simulink model "Diesel_Genset_Test_System"  (Simulink 8.1)
settings: Solver=ode3  SolverMode=SingleTasking  StartTime=0.0  StopTime=150  FixedStep=Ts  RelTol=1e-3
PostLoadFcn:
  | Ts=50e-6;SIM_HIL=0;
InitFcn:
  | Ts=50e-6;SIM_HIL=0;
undefined symbols (not defined in the file): Gen_900kW_external_control, HIL_GenSet, Left, type, V
libraries: powerlib x31, powerlib_extras x24, simulink x10, dspsigops x6, breakers_1ph_3ph x6, rtio_generic_modbus x6, cables_lib x5, rtlab x2, ssn_lib x2, artemis x1, Diesel_Genset_lib x1
(part 2 of 3)

== system Diesel_Genset_Test_System/SM_Master/MODBUS8 ==
  note: S commands:
      | S: 0 , for logic operated relays
      | S: 1 ,  for remotely close the breaker unit
      | S: 2 , for remotely open the breaker unit
  Op_Mode : Inport
  Bus Creator : BusCreator  Inputs=2
  Data Type Conversion1 : DataTypeConversion
  Delay1 : dspsigops/Delay  dly_unit=Samples  delay=lower((3/60)/Ts)  ic_detail=off  dif_ic_for_ch=off  dif_ic_for_dly=off  ic=1  reset_popup=None
  Ground : powerlib/Elements/Ground  LConnTagsString=a
  Index Vector : MultiPortSwitch  DataPortOrder=Zero-based contiguous  DataPortIndices={2,1,0}  zeroidx=on
  SEL_787_Relay : Subsystem
  Three-Phase Parallel RLC Branch : powerlib/Elements/Three-Phase Parallel RLC Branch  LConnTagsString=A|B|C  RConnTagsString=A|B|C  BranchType=R  Resistance=10e6  Inductance=1e-3  Capacitance=1e-6  Measurements=None
  Three-Phase V-I Measurement : powerlib/Measurements/Three-Phase V-I Measurement  VoltageMeasurement=phase-to-ground  SetLabelV=off  LabelV=Vabc  Vpu=off  VpuLL=off  CurrentMeasurement=yes  SetLabelI=off  LabelI=Iabc  Ipu=off  Pbase=100e6  Vbase=500e3  OutputType=Complex  PhasorSimulation=off  PSBequivalent=0
  Three-Phase Breaker : powerlib/Elements/Three-Phase Breaker  InitialState=open  SwitchA=on  SwitchB=on  SwitchC=on  SwitchTimes="[1/60  5/60]"  External=on  BreakerResistance=1e-3  SnubberResistance=0  SnubberCapacitance=0  Measurements=None
  close : Constant
  open : Constant  Value=0
  A : PMIOPort  Tag=PMCPort  Port=1  Side=Left
  B : PMIOPort  Tag=PMCPort  Port=2  Side=Left
  C : PMIOPort  Tag=PMCPort  Port=3  Side=Left
  a : PMIOPort  Tag=PMCPort  Port=4  Side=Right
  b : PMIOPort  Tag=PMCPort  Port=5  Side=Right
  c : PMIOPort  Tag=PMCPort  Port=6  Side=Right
  m : Outport
  wires:
  [m] -> Bus Creator/2  "sel_787"
  SEL_787_Relay/3(m) -> [m]
  Bus Creator/1 -> m/1  "m"
  [Status] -> Bus Creator/1  "Grid_Status"
  Delay1/1 -> [Status], Three-Phase Breaker/1
  Three-Phase V-I Measurement/1 -> [Vabc]
  Three-Phase V-I Measurement/2 -> [Iabc]
  open/1 -> Index Vector/4
  close/1 -> Index Vector/3
  Index Vector/1 -> Data Type Conversion1/1
  Data Type Conversion1/1 -> Delay1/1
  [Iabc] -> SEL_787_Relay/1(Iabc_w1)  "Iabc"
  [Vabc] -> SEL_787_Relay/2(Vabc)  "Vabc"
  SEL_787_Relay/2(Logic_trip) -> Index Vector/2
  Op_Mode/1 -> Index Vector/1
  connections:
  Three-Phase V-I Measurement/RConn1 -- Three-Phase Parallel RLC Branch/RConn1 -- Three-Phase Breaker/LConn1
  Three-Phase V-I Measurement/RConn2 -- Three-Phase Parallel RLC Branch/RConn2 -- Three-Phase Breaker/LConn2
  Three-Phase V-I Measurement/RConn3 -- Three-Phase Parallel RLC Branch/RConn3 -- Three-Phase Breaker/LConn3
  Three-Phase Breaker/RConn2 -- b/RConn1
  Three-Phase Breaker/RConn3 -- c/RConn1
  Three-Phase V-I Measurement/LConn1 -- A/RConn1
  a/RConn1 -- Three-Phase Breaker/RConn1
  C/RConn1 -- Three-Phase V-I Measurement/LConn3
  B/RConn1 -- Three-Phase V-I Measurement/LConn2
  Ground/LConn1 -- Three-Phase Parallel RLC Branch/LConn2 -- Three-Phase Parallel RLC Branch/LConn3 -- Three-Phase Parallel RLC Branch/LConn1

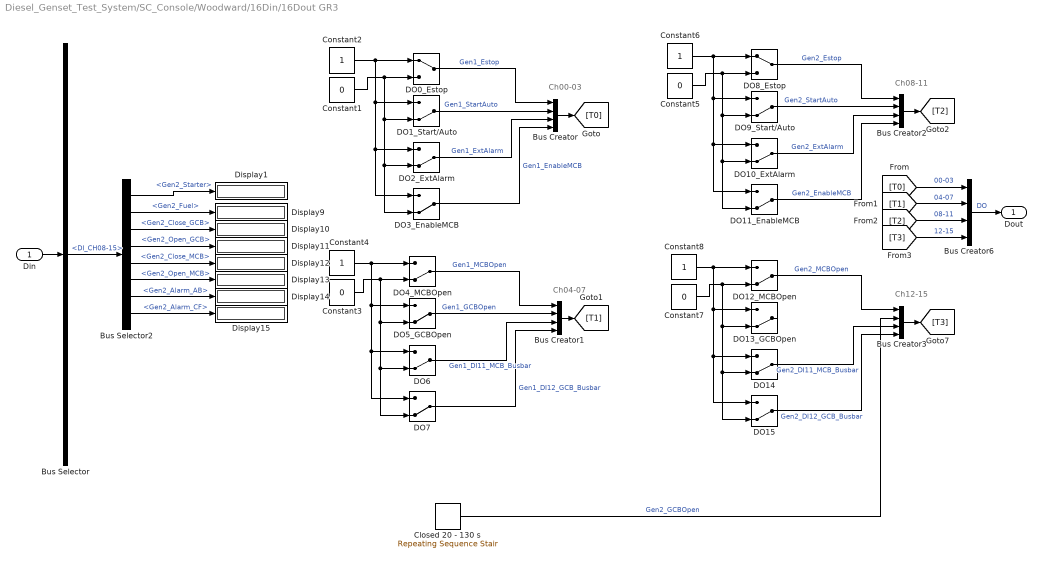
== system Diesel_Genset_Test_System/SC_Console/Woodward/16Din/16Dout GR3 ==
  note: Ch00-03
  note: Ch04-07
  note: Ch08-11
  note: Ch12-15
  Din : Inport
  Bus Creator{,1..3,6} (5 alike) : BusCreator
  Bus Selector : BusSelector  OutputSignals=DIN.DI_CH08-15
  Bus Selector2 : BusSelector  OutputSignals=Gen2_Starter,Gen2_Fuel,Gen2_Close_GCB,Gen2_Open_GCB,Gen2_Close_MCB,Gen2_Open_MCB,Gen2_Alarm_AB,Gen2_Alarm_CF
  Closed 20 - 130 s : simulink/Sources/Repeating Sequence Stair  OutValues=[1 1 1 1 0 0 0 0 0 0 0 0 0 0 0 0 0 0 0 0 0 0 0 0 0 0 1 1 1 1 1 ]  tsamp=[5 Ts]  OutMin=[]  OutMax=[]  OutDataTypeStr=double  OutputDataTypeScalingMode=double  OutDataType=fixdt(0,8)  ConRadixGroup=Best Precision: Vector-wise  OutScaling=2^-12
  Constant{1,3,5,7} (4 alike) : Constant  Value=0
  Constant{2,4,6,8} (4 alike) : Constant
  DO0_Estop : ManualSwitch
  DO10_ExtAlarm : ManualSwitch  CurrentSetting=0
  DO11_EnableMCB : ManualSwitch  CurrentSetting=0
  DO12_MCBOpen : ManualSwitch  CurrentSetting=0
  DO13_GCBOpen : ManualSwitch  CurrentSetting=0
  DO{6..7,14..15} (4 alike) : ManualSwitch  CurrentSetting=0
  DO1_Start/Auto : ManualSwitch  CurrentSetting=0
  DO2_ExtAlarm : ManualSwitch  CurrentSetting=0
  DO3_EnableMCB : ManualSwitch  CurrentSetting=0
  DO4_MCBOpen : ManualSwitch  CurrentSetting=0
  DO5_GCBOpen : ManualSwitch  CurrentSetting=0
  DO8_Estop : ManualSwitch
  DO9_Start/Auto : ManualSwitch  CurrentSetting=0
  Display{1,9..15} (8 alike) : Display
  Dout : Outport
  wires:
  Bus Creator6/1 -> Dout/1  "DO"
  Constant2/1 -> DO0_Estop/1, DO1_Start/Auto/1, DO3_EnableMCB/1, DO2_ExtAlarm/1
  Constant1/1 -> DO0_Estop/2, DO1_Start/Auto/2, DO3_EnableMCB/2, DO2_ExtAlarm/2
  DO0_Estop/1 -> Bus Creator/1  "Gen1_Estop"
  DO1_Start/Auto/1 -> Bus Creator/2  "Gen1_StartAuto"
  DO2_ExtAlarm/1 -> Bus Creator/3  "Gen1_ExtAlarm"
  DO3_EnableMCB/1 -> Bus Creator/4  "Gen1_EnableMCB"
  Constant4/1 -> DO6/1, DO7/1, DO5_GCBOpen/1, DO4_MCBOpen/1
  Constant3/1 -> DO6/2, DO7/2, DO5_GCBOpen/2, DO4_MCBOpen/2
  DO4_MCBOpen/1 -> Bus Creator1/1  "Gen1_MCBOpen"
  DO6/1 -> Bus Creator1/3  "Gen1_DI11_MCB_Busbar"
  DO7/1 -> Bus Creator1/4  "Gen1_DI12_GCB_Busbar"
  Constant6/1 -> DO8_Estop/1, DO9_Start/Auto/1, DO11_EnableMCB/1, DO10_ExtAlarm/1
  Constant5/1 -> DO8_Estop/2, DO9_Start/Auto/2, DO11_EnableMCB/2, DO10_ExtAlarm/2
  DO8_Estop/1 -> Bus Creator2/1  "Gen2_Estop"
  DO9_Start/Auto/1 -> Bus Creator2/2  "Gen2_StartAuto"
  DO10_ExtAlarm/1 -> Bus Creator2/3  "Gen2_ExtAlarm"
  DO11_EnableMCB/1 -> Bus Creator2/4  "Gen2_EnableMCB"
  Constant8/1 -> DO14/1, DO15/1, DO13_GCBOpen/1, DO12_MCBOpen/1
  Constant7/1 -> DO14/2, DO15/2, DO13_GCBOpen/2, DO12_MCBOpen/2
  DO12_MCBOpen/1 -> Bus Creator3/1  "Gen2_MCBOpen"
  DO14/1 -> Bus Creator3/3  "Gen2_DI11_MCB_Busbar"
  DO15/1 -> Bus Creator3/4  "Gen2_DI12_GCB_Busbar"
  Bus Creator/1 -> [T0]
  Bus Creator1/1 -> [T1]
  Bus Creator3/1 -> [T3]
  Bus Creator2/1 -> [T2]
  [T0] -> Bus Creator6/1  "00-03"
  [T1] -> Bus Creator6/2  "04-07"
  [T2] -> Bus Creator6/3  "08-11"
  [T3] -> Bus Creator6/4  "12-15"
  Din/1 -> Bus Selector/1
  Bus Selector/1 -> Bus Selector2/1  "<DI_CH08-15>"
  Bus Selector2/1 -> Display1/1  "<Gen2_Starter>"
  Bus Selector2/2 -> Display9/1  "<Gen2_Fuel>"
  Bus Selector2/3 -> Display10/1  "<Gen2_Close_GCB>"
  Bus Selector2/4 -> Display11/1  "<Gen2_Open_GCB>"
  Bus Selector2/5 -> Display12/1  "<Gen2_Close_MCB>"
  Bus Selector2/6 -> Display13/1  "<Gen2_Open_MCB>"
  Bus Selector2/7 -> Display14/1  "<Gen2_Alarm_AB>"
  Bus Selector2/8 -> Display15/1  "<Gen2_Alarm_CF>"
  DO5_GCBOpen/1 -> Bus Creator1/2  "Gen1_GCBOpen"
  Closed 20 - 130 s/1 -> Bus Creator3/2  "Gen2_GCBOpen"

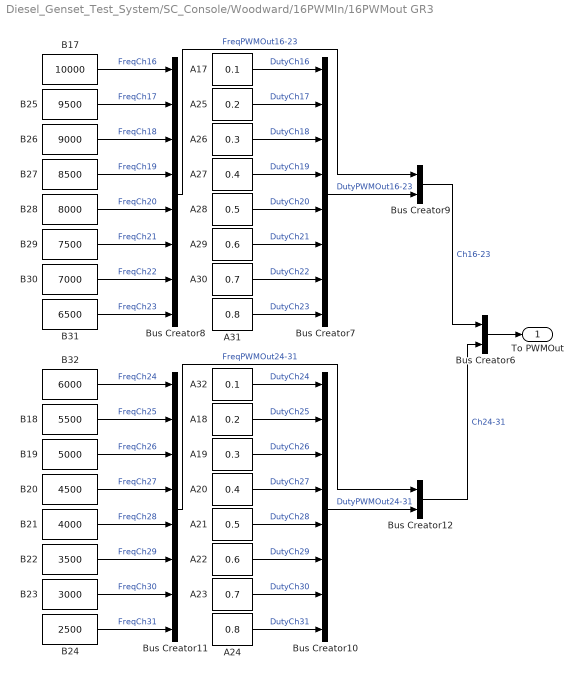
== system Diesel_Genset_Test_System/SC_Console/Woodward/16PWMIn/16PWMout GR3 ==
  A17 : Constant  Value=0.1
  A18 : Constant  Value=0.2
  A19 : Constant  Value=0.3
  A20 : Constant  Value=0.4
  A21 : Constant  Value=0.5
  A22 : Constant  Value=0.6
  A23 : Constant  Value=0.7
  A24 : Constant  Value=0.8
  A25 : Constant  Value=0.2
  A26 : Constant  Value=0.3
  A27 : Constant  Value=0.4
  A28 : Constant  Value=0.5
  A29 : Constant  Value=0.6
  A30 : Constant  Value=0.7
  A31 : Constant  Value=0.8
  A32 : Constant  Value=0.1
  B17 : Constant  Value=10000
  B18 : Constant  Value=5500
  B19 : Constant  Value=5000
  B20 : Constant  Value=4500
  B21 : Constant  Value=4000
  B22 : Constant  Value=3500
  B23 : Constant  Value=3000
  B24 : Constant  Value=2500
  B25 : Constant  Value=9500
  B26 : Constant  Value=9000
  B27 : Constant  Value=8500
  B28 : Constant  Value=8000
  B29 : Constant  Value=7500
  B30 : Constant  Value=7000
  B31 : Constant  Value=6500
  B32 : Constant  Value=6000
  Bus Creator{7..8,10..11} (4 alike) : BusCreator  Inputs=8
  Bus Creator12 : BusCreator  Inputs=2
  Bus Creator6 : BusCreator  Inputs=2
  Bus Creator9 : BusCreator  Inputs=2
  To PWMOut : Outport
  wires:
  Bus Creator6/1 -> To PWMOut/1
  A17/1 -> Bus Creator7/1  "DutyCh16"
  A25/1 -> Bus Creator7/2  "DutyCh17"
  A26/1 -> Bus Creator7/3  "DutyCh18"
  A27/1 -> Bus Creator7/4  "DutyCh19"
  A28/1 -> Bus Creator7/5  "DutyCh20"
  A29/1 -> Bus Creator7/6  "DutyCh21"
  A30/1 -> Bus Creator7/7  "DutyCh22"
  A31/1 -> Bus Creator7/8  "DutyCh23"
  B17/1 -> Bus Creator8/1  "FreqCh16"
  B25/1 -> Bus Creator8/2  "FreqCh17"
  B26/1 -> Bus Creator8/3  "FreqCh18"
  B27/1 -> Bus Creator8/4  "FreqCh19"
  B28/1 -> Bus Creator8/5  "FreqCh20"
  B29/1 -> Bus Creator8/6  "FreqCh21"
  B30/1 -> Bus Creator8/7  "FreqCh22"
  B31/1 -> Bus Creator8/8  "FreqCh23"
  Bus Creator7/1 -> Bus Creator9/2  "DutyPWMOut16-23"
  Bus Creator8/1 -> Bus Creator9/1  "FreqPWMOut16-23"
  A32/1 -> Bus Creator10/1  "DutyCh24"
  A18/1 -> Bus Creator10/2  "DutyCh25"
  A19/1 -> Bus Creator10/3  "DutyCh26"
  A20/1 -> Bus Creator10/4  "DutyCh27"
  A21/1 -> Bus Creator10/5  "DutyCh28"
  A22/1 -> Bus Creator10/6  "DutyCh29"
  A23/1 -> Bus Creator10/7  "DutyCh30"
  A24/1 -> Bus Creator10/8  "DutyCh31"
  B32/1 -> Bus Creator11/1  "FreqCh24"
  B18/1 -> Bus Creator11/2  "FreqCh25"
  B19/1 -> Bus Creator11/3  "FreqCh26"
  B20/1 -> Bus Creator11/4  "FreqCh27"
  B21/1 -> Bus Creator11/5  "FreqCh28"
  B22/1 -> Bus Creator11/6  "FreqCh29"
  B23/1 -> Bus Creator11/7  "FreqCh30"
  B24/1 -> Bus Creator11/8  "FreqCh31"
  Bus Creator10/1 -> Bus Creator12/2  "DutyPWMOut24-31"
  Bus Creator11/1 -> Bus Creator12/1  "FreqPWMOut24-31"
  Bus Creator12/1 -> Bus Creator6/2  "Ch24-31"
  Bus Creator9/1 -> Bus Creator6/1  "Ch16-23"

== system Diesel_Genset_Test_System/SC_Console/Woodward/16TSDIn/16 TSDOut GR3 ==
  Bus Creator1 : BusCreator  Inputs=3
  Din/Dout ch16-23 : Subsystem
  Din/Dout ch24-31 : Subsystem
  Dout state ctrl : Subsystem
  TSDout : Outport
  wires:
  Din/Dout ch24-31/1(Out1) -> Bus Creator1/2  "times CH24-31"
  Din/Dout ch16-23/1(Out1) -> Bus Creator1/1  "times CH16-23"
  Dout state ctrl/1(Event State OUT) -> Bus Creator1/3  "states"
  Bus Creator1/1 -> TSDout/1

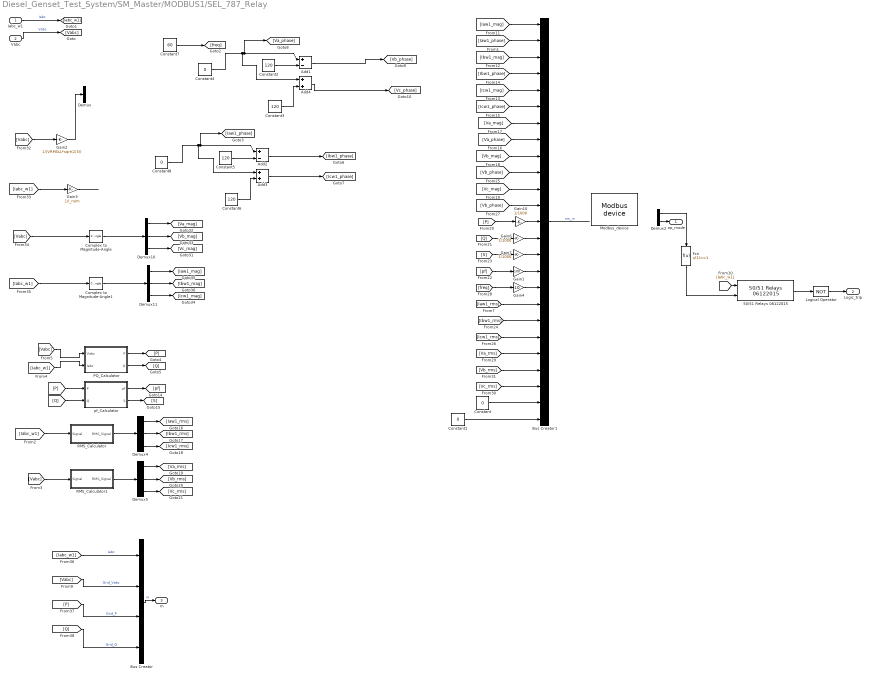
== system Diesel_Genset_Test_System/SM_Master/MODBUS1/SEL_787_Relay ==
  Iabc_w1 : Inport
  Vabc : Inport  Port=2
  50/51 Relays 06122015 : breakers_1ph_3ph/50//51 Relays 06122015  TOC=TOC  IOC=IOC  Ts=Ts
  Add1 : Sum  Inputs=+-
  Add2 : Sum  Inputs=+-
  Add3 : Sum
  Add4 : Sum
  Bus Creator : BusCreator
  Bus Creator1 : BusCreator  Inputs=25
  Complex to Magnitude-Angle : ComplexToMagnitudeAngle  Output=Magnitude
  Complex to Magnitude-Angle1 : ComplexToMagnitudeAngle  Output=Magnitude
  Constant{,1,4,8} (4 alike) : Constant  Value=0
  Constant{2..3,5..6} (4 alike) : Constant  Value=120
  Constant7 : Constant  Value=60
  Demux{,4..5,10..11} (5 alike) : Demux  Outputs=3
  Demux2 : Demux  Outputs=2
  Fcn : Fcn  Expr=u(1)==1
  Gain1 : Gain  Gain=100
  Gain10 : Gain  Gain=1/1000
  Gain2 : Gain  Gain=1/(VRMSLL*sqrt(2/3))
  Gain3 : Gain  Gain=1/I_nom
  Gain4 : Gain  Gain=10
  Gain6 : Gain  Gain=1/1000
  Gain7 : Gain  Gain=1/1000
  Logical Operator : Logic  Operator=NOT  AllPortsSameDT=off  OutDataTypeStr=boolean
  Modbus_device : rtio_generic_modbus/Modbus device  conf_name=none  conf_name_mask=relay_slave_cfg1.xls  sample_time=Ts
  PQ_Calculator : Subsystem
  RMS_Calculator : Subsystem
  RMS_Calculator1 : Subsystem
  pf_Calculator : Subsystem
  op_mode : Outport
  Logic_trip : Outport  Port=2
  m : Outport  Port=3
  wires:
  Gain4/1 -> Bus Creator1/17
  Gain1/1 -> Bus Creator1/16
  [pf] -> Gain1/1
  [freq] -> Gain4/1
  Constant4/1 -> Add4/1, [Va_phase], Add1/1
  Add4/1 -> [Vc_phase]
  Add1/1 -> [Vb_phase]
  Constant3/1 -> Add4/2
  Constant2/1 -> Add1/2
  Constant8/1 -> Add3/1, [Iaw1_phase], Add2/1
  Add3/1 -> [Icw1_phase]
  Add2/1 -> [Ibw1_phase]
  Constant6/1 -> Add3/2
  Constant5/1 -> Add2/2
  Constant7/1 -> [freq]
  pf_Calculator/2(S) -> [S]
  Bus Creator1/1 -> ?  "sm_in"
  ? -> Demux2/1
  [Q] -> Bus Creator/4  "Grid_Q"
  [P] -> Bus Creator/3  "Grid_P"
  [Vabc] -> Bus Creator/2  "Grid_Vabc"
  [Iabc_w1] -> Bus Creator/1  "Iabc"
  Bus Creator/1 -> m/1  "m"
  Iabc_w1/1 -> [Iabc_w1]  "Iabc"
  Vabc/1 -> [Vabc]  "Vabc"
  [Vabc] -> PQ_Calculator/1(Vabc)
  [Iabc_w1] -> PQ_Calculator/2(Iabc)
  [Iaw1_mag] -> Bus Creator1/1
  [P] -> Gain10/1
  [Q] -> Gain6/1
  [S] -> Gain7/1
  pf_Calculator/1(pf) -> [pf]
  [P] -> pf_Calculator/1(P)
  [Q] -> pf_Calculator/2(Q)
  PQ_Calculator/1(P) -> [P]
  PQ_Calculator/2(Q) -> [Q]
  [Iabc_w1] -> RMS_Calculator/1(Signal)
  [Vabc] -> RMS_Calculator1/1(Signal)
  RMS_Calculator/1(RMS_Signal) -> Demux4/1
  RMS_Calculator1/1(RMS_Signal) -> Demux5/1
  Demux4/3 -> [Icw1_rms]
  Demux4/2 -> [Ibw1_rms]
  Demux4/1 -> [Iaw1_rms]
  Demux5/1 -> [Va_rms]
  Demux5/2 -> [Vb_rms]
  Demux5/3 -> [Vc_rms]
  Demux2/1 -> Fcn/1
  Fcn/1 -> 50/51 Relays 06122015/2
  [Iabc_w1] -> 50/51 Relays 06122015/1
  50/51 Relays 06122015/1 -> Logical Operator/1
  [Ibw1_mag] -> Bus Creator1/3
  [Icw1_mag] -> Bus Creator1/5
  [Va_mag] -> Bus Creator1/7
  [Vb_mag] -> Bus Creator1/9
  [Vc_mag] -> Bus Creator1/11
  Gain10/1 -> Bus Creator1/13
  Gain6/1 -> Bus Creator1/14
  Gain7/1 -> Bus Creator1/15
  [Iaw1_rms] -> Bus Creator1/18
  [Icw1_rms] -> Bus Creator1/20
  [Ibw1_rms] -> Bus Creator1/19
  [Va_rms] -> Bus Creator1/21
  [Vb_rms] -> Bus Creator1/22
  [Vc_rms] -> Bus Creator1/23
  Logical Operator/1 -> Logic_trip/1
  Demux2/2 -> op_mode/1
  [Iaw1_phase] -> Bus Creator1/2
  [Ibw1_phase] -> Bus Creator1/4
  [Icw1_phase] -> Bus Creator1/6
  [Va_phase] -> Bus Creator1/8
  [Vb_phase] -> Bus Creator1/10
  [Vb_phase] -> Bus Creator1/12
  Constant/1 -> Bus Creator1/24
  Constant1/1 -> Bus Creator1/25
  [Vabc] -> Gain2/1
  Gain2/1 -> Demux/1
  [Iabc_w1] -> Gain3/1
  Gain3/1 -> ?
  Demux10/1 -> [Va_mag]
  Demux10/2 -> [Vb_mag]
  Demux10/3 -> [Vc_mag]
  Complex to Magnitude-Angle/1 -> Demux10/1
  [Vabc] -> Complex to Magnitude-Angle/1
  Complex to Magnitude-Angle1/1 -> Demux11/1
  [Iabc_w1] -> Complex to Magnitude-Angle1/1
  Demux11/1 -> [Iaw1_mag]
  Demux11/2 -> [Ibw1_mag]
  Demux11/3 -> [Icw1_mag]

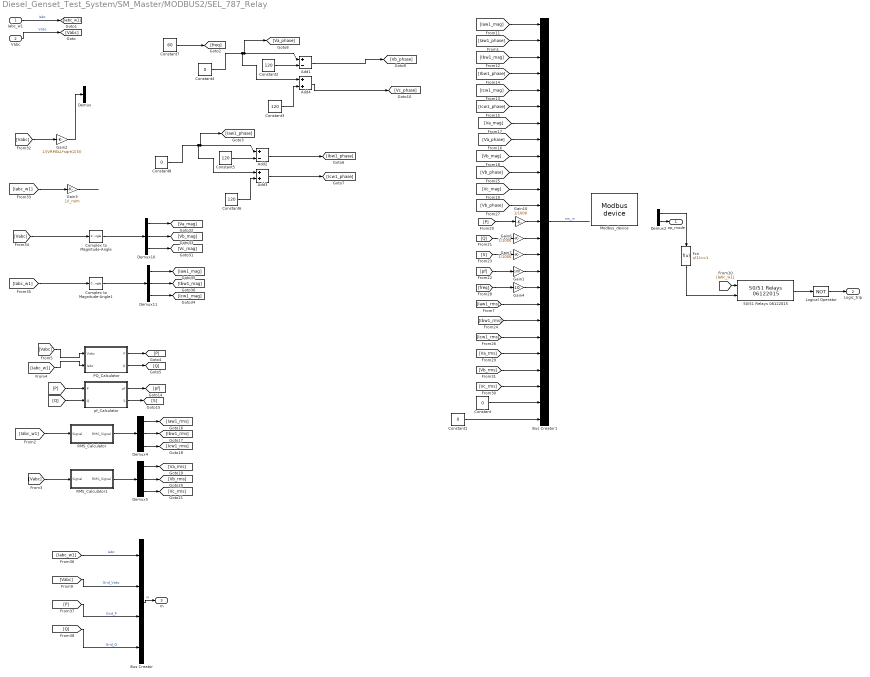
== system Diesel_Genset_Test_System/SM_Master/MODBUS2/SEL_787_Relay ==
  Iabc_w1 : Inport
  Vabc : Inport  Port=2
  50/51 Relays 06122015 : breakers_1ph_3ph/50//51 Relays 06122015  TOC=TOC  IOC=IOC  Ts=Ts
  Add1 : Sum  Inputs=+-
  Add2 : Sum  Inputs=+-
  Add3 : Sum
  Add4 : Sum
  Bus Creator : BusCreator
  Bus Creator1 : BusCreator  Inputs=25
  Complex to Magnitude-Angle : ComplexToMagnitudeAngle  Output=Magnitude
  Complex to Magnitude-Angle1 : ComplexToMagnitudeAngle  Output=Magnitude
  Constant{,1,4,8} (4 alike) : Constant  Value=0
  Constant{2..3,5..6} (4 alike) : Constant  Value=120
  Constant7 : Constant  Value=60
  Demux{,4..5,10..11} (5 alike) : Demux  Outputs=3
  Demux2 : Demux  Outputs=2
  Fcn : Fcn  Expr=u(1)==1
  Gain1 : Gain  Gain=100
  Gain10 : Gain  Gain=1/1000
  Gain2 : Gain  Gain=1/(VRMSLL*sqrt(2/3))
  Gain3 : Gain  Gain=1/I_nom
  Gain4 : Gain  Gain=10
  Gain6 : Gain  Gain=1/1000
  Gain7 : Gain  Gain=1/1000
  Logical Operator : Logic  Operator=NOT  AllPortsSameDT=off  OutDataTypeStr=boolean
  Modbus_device : rtio_generic_modbus/Modbus device  conf_name=none  conf_name_mask=relay_slave_cfg2.xls  sample_time=Ts
  PQ_Calculator : Subsystem
  RMS_Calculator : Subsystem
  RMS_Calculator1 : Subsystem
  pf_Calculator : Subsystem
  op_mode : Outport
  Logic_trip : Outport  Port=2
  m : Outport  Port=3
  wires:
  Gain4/1 -> Bus Creator1/17
  Gain1/1 -> Bus Creator1/16
  [pf] -> Gain1/1
  [freq] -> Gain4/1
  Constant4/1 -> Add4/1, [Va_phase], Add1/1
  Add4/1 -> [Vc_phase]
  Add1/1 -> [Vb_phase]
  Constant3/1 -> Add4/2
  Constant2/1 -> Add1/2
  Constant8/1 -> Add3/1, [Iaw1_phase], Add2/1
  Add3/1 -> [Icw1_phase]
  Add2/1 -> [Ibw1_phase]
  Constant6/1 -> Add3/2
  Constant5/1 -> Add2/2
  Constant7/1 -> [freq]
  pf_Calculator/2(S) -> [S]
  Bus Creator1/1 -> ?  "sm_in"
  ? -> Demux2/1
  [Q] -> Bus Creator/4  "Grid_Q"
  [P] -> Bus Creator/3  "Grid_P"
  [Vabc] -> Bus Creator/2  "Grid_Vabc"
  [Iabc_w1] -> Bus Creator/1  "Iabc"
  Bus Creator/1 -> m/1  "m"
  Iabc_w1/1 -> [Iabc_w1]  "Iabc"
  Vabc/1 -> [Vabc]  "Vabc"
  [Vabc] -> PQ_Calculator/1(Vabc)
  [Iabc_w1] -> PQ_Calculator/2(Iabc)
  [Iaw1_mag] -> Bus Creator1/1
  [P] -> Gain10/1
  [Q] -> Gain6/1
  [S] -> Gain7/1
  pf_Calculator/1(pf) -> [pf]
  [P] -> pf_Calculator/1(P)
  [Q] -> pf_Calculator/2(Q)
  PQ_Calculator/1(P) -> [P]
  PQ_Calculator/2(Q) -> [Q]
  [Iabc_w1] -> RMS_Calculator/1(Signal)
  [Vabc] -> RMS_Calculator1/1(Signal)
  RMS_Calculator/1(RMS_Signal) -> Demux4/1
  RMS_Calculator1/1(RMS_Signal) -> Demux5/1
  Demux4/3 -> [Icw1_rms]
  Demux4/2 -> [Ibw1_rms]
  Demux4/1 -> [Iaw1_rms]
  Demux5/1 -> [Va_rms]
  Demux5/2 -> [Vb_rms]
  Demux5/3 -> [Vc_rms]
  Demux2/1 -> Fcn/1
  Fcn/1 -> 50/51 Relays 06122015/2
  [Iabc_w1] -> 50/51 Relays 06122015/1
  50/51 Relays 06122015/1 -> Logical Operator/1
  [Ibw1_mag] -> Bus Creator1/3
  [Icw1_mag] -> Bus Creator1/5
  [Va_mag] -> Bus Creator1/7
  [Vb_mag] -> Bus Creator1/9
  [Vc_mag] -> Bus Creator1/11
  Gain10/1 -> Bus Creator1/13
  Gain6/1 -> Bus Creator1/14
  Gain7/1 -> Bus Creator1/15
  [Iaw1_rms] -> Bus Creator1/18
  [Icw1_rms] -> Bus Creator1/20
  [Ibw1_rms] -> Bus Creator1/19
  [Va_rms] -> Bus Creator1/21
  [Vb_rms] -> Bus Creator1/22
  [Vc_rms] -> Bus Creator1/23
  Logical Operator/1 -> Logic_trip/1
  Demux2/2 -> op_mode/1
  [Iaw1_phase] -> Bus Creator1/2
  [Ibw1_phase] -> Bus Creator1/4
  [Icw1_phase] -> Bus Creator1/6
  [Va_phase] -> Bus Creator1/8
  [Vb_phase] -> Bus Creator1/10
  [Vb_phase] -> Bus Creator1/12
  Constant/1 -> Bus Creator1/24
  Constant1/1 -> Bus Creator1/25
  [Vabc] -> Gain2/1
  Gain2/1 -> Demux/1
  [Iabc_w1] -> Gain3/1
  Gain3/1 -> ?
  Demux10/1 -> [Va_mag]
  Demux10/2 -> [Vb_mag]
  Demux10/3 -> [Vc_mag]
  Complex to Magnitude-Angle/1 -> Demux10/1
  [Vabc] -> Complex to Magnitude-Angle/1
  Complex to Magnitude-Angle1/1 -> Demux11/1
  [Iabc_w1] -> Complex to Magnitude-Angle1/1
  Demux11/1 -> [Iaw1_mag]
  Demux11/2 -> [Ibw1_mag]
  Demux11/3 -> [Icw1_mag]

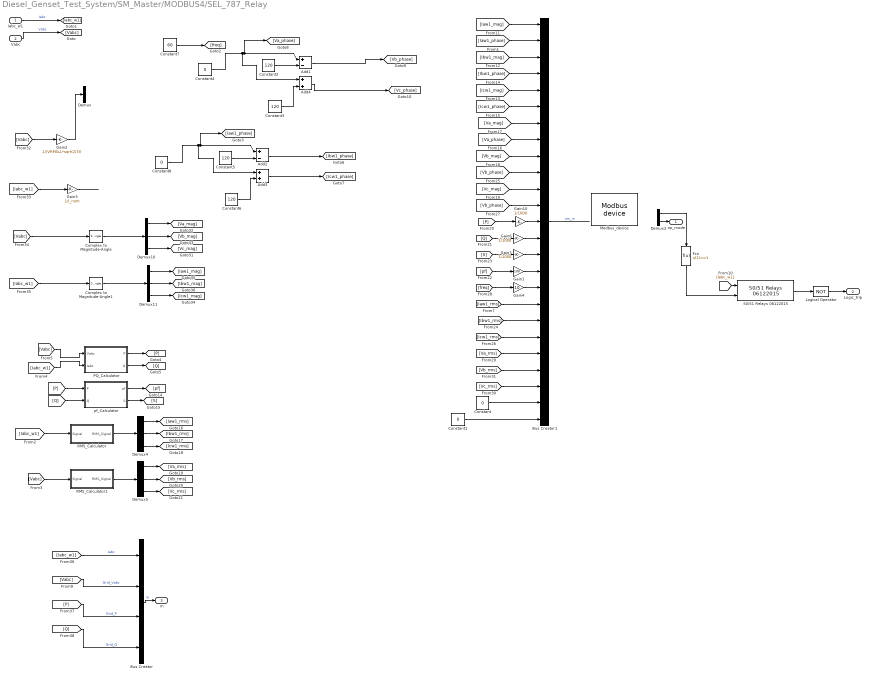
== system Diesel_Genset_Test_System/SM_Master/MODBUS4/SEL_787_Relay ==
  Iabc_w1 : Inport
  Vabc : Inport  Port=2
  50/51 Relays 06122015 : breakers_1ph_3ph/50//51 Relays 06122015  TOC=TOC  IOC=IOC  Ts=Ts
  Add1 : Sum  Inputs=+-
  Add2 : Sum  Inputs=+-
  Add3 : Sum
  Add4 : Sum
  Bus Creator : BusCreator
  Bus Creator1 : BusCreator  Inputs=25
  Complex to Magnitude-Angle : ComplexToMagnitudeAngle  Output=Magnitude
  Complex to Magnitude-Angle1 : ComplexToMagnitudeAngle  Output=Magnitude
  Constant{,1,4,8} (4 alike) : Constant  Value=0
  Constant{2..3,5..6} (4 alike) : Constant  Value=120
  Constant7 : Constant  Value=60
  Demux{,4..5,10..11} (5 alike) : Demux  Outputs=3
  Demux2 : Demux  Outputs=2
  Fcn : Fcn  Expr=u(1)==1
  Gain1 : Gain  Gain=100
  Gain10 : Gain  Gain=1/1000
  Gain2 : Gain  Gain=1/(VRMSLL*sqrt(2/3))
  Gain3 : Gain  Gain=1/I_nom
  Gain4 : Gain  Gain=10
  Gain6 : Gain  Gain=1/1000
  Gain7 : Gain  Gain=1/1000
  Logical Operator : Logic  Operator=NOT  AllPortsSameDT=off  OutDataTypeStr=boolean
  Modbus_device : rtio_generic_modbus/Modbus device  conf_name=none  conf_name_mask=relay_slave_cfg4.xls  sample_time=Ts
  PQ_Calculator : Subsystem
  RMS_Calculator : Subsystem
  RMS_Calculator1 : Subsystem
  pf_Calculator : Subsystem
  op_mode : Outport
  Logic_trip : Outport  Port=2
  m : Outport  Port=3
  wires:
  Gain4/1 -> Bus Creator1/17
  Gain1/1 -> Bus Creator1/16
  [pf] -> Gain1/1
  [freq] -> Gain4/1
  Constant4/1 -> Add4/1, [Va_phase], Add1/1
  Add4/1 -> [Vc_phase]
  Add1/1 -> [Vb_phase]
  Constant3/1 -> Add4/2
  Constant2/1 -> Add1/2
  Constant8/1 -> Add3/1, [Iaw1_phase], Add2/1
  Add3/1 -> [Icw1_phase]
  Add2/1 -> [Ibw1_phase]
  Constant6/1 -> Add3/2
  Constant5/1 -> Add2/2
  Constant7/1 -> [freq]
  pf_Calculator/2(S) -> [S]
  Bus Creator1/1 -> ?  "sm_in"
  ? -> Demux2/1
  [Q] -> Bus Creator/4  "Grid_Q"
  [P] -> Bus Creator/3  "Grid_P"
  [Vabc] -> Bus Creator/2  "Grid_Vabc"
  [Iabc_w1] -> Bus Creator/1  "Iabc"
  Bus Creator/1 -> m/1  "m"
  Iabc_w1/1 -> [Iabc_w1]  "Iabc"
  Vabc/1 -> [Vabc]  "Vabc"
  [Vabc] -> PQ_Calculator/1(Vabc)
  [Iabc_w1] -> PQ_Calculator/2(Iabc)
  [Iaw1_mag] -> Bus Creator1/1
  [P] -> Gain10/1
  [Q] -> Gain6/1
  [S] -> Gain7/1
  pf_Calculator/1(pf) -> [pf]
  [P] -> pf_Calculator/1(P)
  [Q] -> pf_Calculator/2(Q)
  PQ_Calculator/1(P) -> [P]
  PQ_Calculator/2(Q) -> [Q]
  [Iabc_w1] -> RMS_Calculator/1(Signal)
  [Vabc] -> RMS_Calculator1/1(Signal)
  RMS_Calculator/1(RMS_Signal) -> Demux4/1
  RMS_Calculator1/1(RMS_Signal) -> Demux5/1
  Demux4/3 -> [Icw1_rms]
  Demux4/2 -> [Ibw1_rms]
  Demux4/1 -> [Iaw1_rms]
  Demux5/1 -> [Va_rms]
  Demux5/2 -> [Vb_rms]
  Demux5/3 -> [Vc_rms]
  Demux2/1 -> Fcn/1
  Fcn/1 -> 50/51 Relays 06122015/2
  [Iabc_w1] -> 50/51 Relays 06122015/1
  50/51 Relays 06122015/1 -> Logical Operator/1
  [Ibw1_mag] -> Bus Creator1/3
  [Icw1_mag] -> Bus Creator1/5
  [Va_mag] -> Bus Creator1/7
  [Vb_mag] -> Bus Creator1/9
  [Vc_mag] -> Bus Creator1/11
  Gain10/1 -> Bus Creator1/13
  Gain6/1 -> Bus Creator1/14
  Gain7/1 -> Bus Creator1/15
  [Iaw1_rms] -> Bus Creator1/18
  [Icw1_rms] -> Bus Creator1/20
  [Ibw1_rms] -> Bus Creator1/19
  [Va_rms] -> Bus Creator1/21
  [Vb_rms] -> Bus Creator1/22
  [Vc_rms] -> Bus Creator1/23
  Logical Operator/1 -> Logic_trip/1
  Demux2/2 -> op_mode/1
  [Iaw1_phase] -> Bus Creator1/2
  [Ibw1_phase] -> Bus Creator1/4
  [Icw1_phase] -> Bus Creator1/6
  [Va_phase] -> Bus Creator1/8
  [Vb_phase] -> Bus Creator1/10
  [Vb_phase] -> Bus Creator1/12
  Constant/1 -> Bus Creator1/24
  Constant1/1 -> Bus Creator1/25
  [Vabc] -> Gain2/1
  Gain2/1 -> Demux/1
  [Iabc_w1] -> Gain3/1
  Gain3/1 -> ?
  Demux10/1 -> [Va_mag]
  Demux10/2 -> [Vb_mag]
  Demux10/3 -> [Vc_mag]
  Complex to Magnitude-Angle/1 -> Demux10/1
  [Vabc] -> Complex to Magnitude-Angle/1
  Complex to Magnitude-Angle1/1 -> Demux11/1
  [Iabc_w1] -> Complex to Magnitude-Angle1/1
  Demux11/1 -> [Iaw1_mag]
  Demux11/2 -> [Ibw1_mag]
  Demux11/3 -> [Icw1_mag]

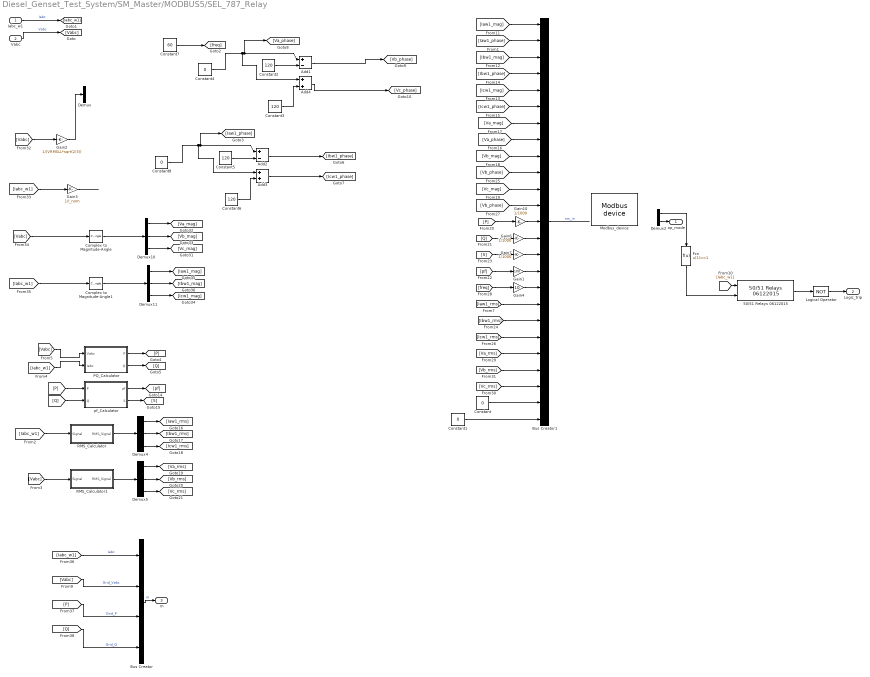
== system Diesel_Genset_Test_System/SM_Master/MODBUS5/SEL_787_Relay ==
  Iabc_w1 : Inport
  Vabc : Inport  Port=2
  50/51 Relays 06122015 : breakers_1ph_3ph/50//51 Relays 06122015  TOC=TOC  IOC=IOC  Ts=Ts
  Add1 : Sum  Inputs=+-
  Add2 : Sum  Inputs=+-
  Add3 : Sum
  Add4 : Sum
  Bus Creator : BusCreator
  Bus Creator1 : BusCreator  Inputs=25
  Complex to Magnitude-Angle : ComplexToMagnitudeAngle  Output=Magnitude
  Complex to Magnitude-Angle1 : ComplexToMagnitudeAngle  Output=Magnitude
  Constant{,1,4,8} (4 alike) : Constant  Value=0
  Constant{2..3,5..6} (4 alike) : Constant  Value=120
  Constant7 : Constant  Value=60
  Demux{,4..5,10..11} (5 alike) : Demux  Outputs=3
  Demux2 : Demux  Outputs=2
  Fcn : Fcn  Expr=u(1)==1
  Gain1 : Gain  Gain=100
  Gain10 : Gain  Gain=1/1000
  Gain2 : Gain  Gain=1/(VRMSLL*sqrt(2/3))
  Gain3 : Gain  Gain=1/I_nom
  Gain4 : Gain  Gain=10
  Gain6 : Gain  Gain=1/1000
  Gain7 : Gain  Gain=1/1000
  Logical Operator : Logic  Operator=NOT  AllPortsSameDT=off  OutDataTypeStr=boolean
  Modbus_device : rtio_generic_modbus/Modbus device  conf_name=none  conf_name_mask=relay_slave_cfg5.xls  sample_time=Ts
  PQ_Calculator : Subsystem
  RMS_Calculator : Subsystem
  RMS_Calculator1 : Subsystem
  pf_Calculator : Subsystem
  op_mode : Outport
  Logic_trip : Outport  Port=2
  m : Outport  Port=3
  wires:
  Gain4/1 -> Bus Creator1/17
  Gain1/1 -> Bus Creator1/16
  [pf] -> Gain1/1
  [freq] -> Gain4/1
  Constant4/1 -> Add4/1, [Va_phase], Add1/1
  Add4/1 -> [Vc_phase]
  Add1/1 -> [Vb_phase]
  Constant3/1 -> Add4/2
  Constant2/1 -> Add1/2
  Constant8/1 -> Add3/1, [Iaw1_phase], Add2/1
  Add3/1 -> [Icw1_phase]
  Add2/1 -> [Ibw1_phase]
  Constant6/1 -> Add3/2
  Constant5/1 -> Add2/2
  Constant7/1 -> [freq]
  pf_Calculator/2(S) -> [S]
  Bus Creator1/1 -> ?  "sm_in"
  ? -> Demux2/1
  [Q] -> Bus Creator/4  "Grid_Q"
  [P] -> Bus Creator/3  "Grid_P"
  [Vabc] -> Bus Creator/2  "Grid_Vabc"
  [Iabc_w1] -> Bus Creator/1  "Iabc"
  Bus Creator/1 -> m/1  "m"
  Iabc_w1/1 -> [Iabc_w1]  "Iabc"
  Vabc/1 -> [Vabc]  "Vabc"
  [Vabc] -> PQ_Calculator/1(Vabc)
  [Iabc_w1] -> PQ_Calculator/2(Iabc)
  [Iaw1_mag] -> Bus Creator1/1
  [P] -> Gain10/1
  [Q] -> Gain6/1
  [S] -> Gain7/1
  pf_Calculator/1(pf) -> [pf]
  [P] -> pf_Calculator/1(P)
  [Q] -> pf_Calculator/2(Q)
  PQ_Calculator/1(P) -> [P]
  PQ_Calculator/2(Q) -> [Q]
  [Iabc_w1] -> RMS_Calculator/1(Signal)
  [Vabc] -> RMS_Calculator1/1(Signal)
  RMS_Calculator/1(RMS_Signal) -> Demux4/1
  RMS_Calculator1/1(RMS_Signal) -> Demux5/1
  Demux4/3 -> [Icw1_rms]
  Demux4/2 -> [Ibw1_rms]
  Demux4/1 -> [Iaw1_rms]
  Demux5/1 -> [Va_rms]
  Demux5/2 -> [Vb_rms]
  Demux5/3 -> [Vc_rms]
  Demux2/1 -> Fcn/1
  Fcn/1 -> 50/51 Relays 06122015/2
  [Iabc_w1] -> 50/51 Relays 06122015/1
  50/51 Relays 06122015/1 -> Logical Operator/1
  [Ibw1_mag] -> Bus Creator1/3
  [Icw1_mag] -> Bus Creator1/5
  [Va_mag] -> Bus Creator1/7
  [Vb_mag] -> Bus Creator1/9
  [Vc_mag] -> Bus Creator1/11
  Gain10/1 -> Bus Creator1/13
  Gain6/1 -> Bus Creator1/14
  Gain7/1 -> Bus Creator1/15
  [Iaw1_rms] -> Bus Creator1/18
  [Icw1_rms] -> Bus Creator1/20
  [Ibw1_rms] -> Bus Creator1/19
  [Va_rms] -> Bus Creator1/21
  [Vb_rms] -> Bus Creator1/22
  [Vc_rms] -> Bus Creator1/23
  Logical Operator/1 -> Logic_trip/1
  Demux2/2 -> op_mode/1
  [Iaw1_phase] -> Bus Creator1/2
  [Ibw1_phase] -> Bus Creator1/4
  [Icw1_phase] -> Bus Creator1/6
  [Va_phase] -> Bus Creator1/8
  [Vb_phase] -> Bus Creator1/10
  [Vb_phase] -> Bus Creator1/12
  Constant/1 -> Bus Creator1/24
  Constant1/1 -> Bus Creator1/25
  [Vabc] -> Gain2/1
  Gain2/1 -> Demux/1
  [Iabc_w1] -> Gain3/1
  Gain3/1 -> ?
  Demux10/1 -> [Va_mag]
  Demux10/2 -> [Vb_mag]
  Demux10/3 -> [Vc_mag]
  Complex to Magnitude-Angle/1 -> Demux10/1
  [Vabc] -> Complex to Magnitude-Angle/1
  Complex to Magnitude-Angle1/1 -> Demux11/1
  [Iabc_w1] -> Complex to Magnitude-Angle1/1
  Demux11/1 -> [Iaw1_mag]
  Demux11/2 -> [Ibw1_mag]
  Demux11/3 -> [Icw1_mag]

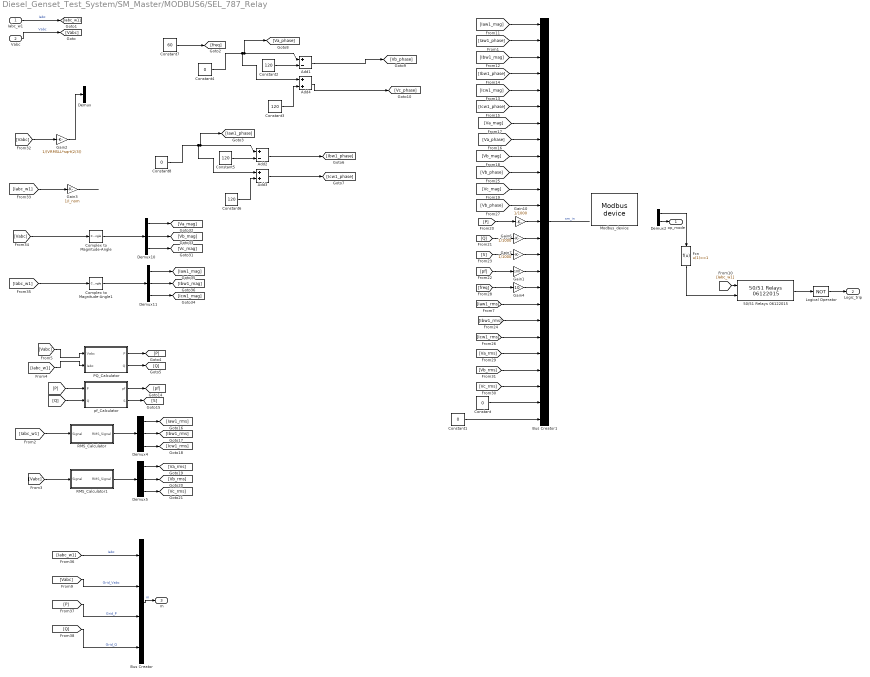
== system Diesel_Genset_Test_System/SM_Master/MODBUS6/SEL_787_Relay ==
  Iabc_w1 : Inport
  Vabc : Inport  Port=2
  50/51 Relays 06122015 : breakers_1ph_3ph/50//51 Relays 06122015  TOC=TOC  IOC=IOC  Ts=Ts
  Add1 : Sum  Inputs=+-
  Add2 : Sum  Inputs=+-
  Add3 : Sum
  Add4 : Sum
  Bus Creator : BusCreator
  Bus Creator1 : BusCreator  Inputs=25
  Complex to Magnitude-Angle : ComplexToMagnitudeAngle  Output=Magnitude
  Complex to Magnitude-Angle1 : ComplexToMagnitudeAngle  Output=Magnitude
  Constant{,1,4,8} (4 alike) : Constant  Value=0
  Constant{2..3,5..6} (4 alike) : Constant  Value=120
  Constant7 : Constant  Value=60
  Demux{,4..5,10..11} (5 alike) : Demux  Outputs=3
  Demux2 : Demux  Outputs=2
  Fcn : Fcn  Expr=u(1)==1
  Gain1 : Gain  Gain=100
  Gain10 : Gain  Gain=1/1000
  Gain2 : Gain  Gain=1/(VRMSLL*sqrt(2/3))
  Gain3 : Gain  Gain=1/I_nom
  Gain4 : Gain  Gain=10
  Gain6 : Gain  Gain=1/1000
  Gain7 : Gain  Gain=1/1000
  Logical Operator : Logic  Operator=NOT  AllPortsSameDT=off  OutDataTypeStr=boolean
  Modbus_device : rtio_generic_modbus/Modbus device  conf_name=none  conf_name_mask=relay_slave_cfg5.xls  sample_time=Ts
  PQ_Calculator : Subsystem
  RMS_Calculator : Subsystem
  RMS_Calculator1 : Subsystem
  pf_Calculator : Subsystem
  op_mode : Outport
  Logic_trip : Outport  Port=2
  m : Outport  Port=3
  wires:
  Gain4/1 -> Bus Creator1/17
  Gain1/1 -> Bus Creator1/16
  [pf] -> Gain1/1
  [freq] -> Gain4/1
  Constant4/1 -> Add4/1, [Va_phase], Add1/1
  Add4/1 -> [Vc_phase]
  Add1/1 -> [Vb_phase]
  Constant3/1 -> Add4/2
  Constant2/1 -> Add1/2
  Constant8/1 -> Add3/1, [Iaw1_phase], Add2/1
  Add3/1 -> [Icw1_phase]
  Add2/1 -> [Ibw1_phase]
  Constant6/1 -> Add3/2
  Constant5/1 -> Add2/2
  Constant7/1 -> [freq]
  pf_Calculator/2(S) -> [S]
  Bus Creator1/1 -> ?  "sm_in"
  ? -> Demux2/1
  [Q] -> Bus Creator/4  "Grid_Q"
  [P] -> Bus Creator/3  "Grid_P"
  [Vabc] -> Bus Creator/2  "Grid_Vabc"
  [Iabc_w1] -> Bus Creator/1  "Iabc"
  Bus Creator/1 -> m/1  "m"
  Iabc_w1/1 -> [Iabc_w1]  "Iabc"
  Vabc/1 -> [Vabc]  "Vabc"
  [Vabc] -> PQ_Calculator/1(Vabc)
  [Iabc_w1] -> PQ_Calculator/2(Iabc)
  [Iaw1_mag] -> Bus Creator1/1
  [P] -> Gain10/1
  [Q] -> Gain6/1
  [S] -> Gain7/1
  pf_Calculator/1(pf) -> [pf]
  [P] -> pf_Calculator/1(P)
  [Q] -> pf_Calculator/2(Q)
  PQ_Calculator/1(P) -> [P]
  PQ_Calculator/2(Q) -> [Q]
  [Iabc_w1] -> RMS_Calculator/1(Signal)
  [Vabc] -> RMS_Calculator1/1(Signal)
  RMS_Calculator/1(RMS_Signal) -> Demux4/1
  RMS_Calculator1/1(RMS_Signal) -> Demux5/1
  Demux4/3 -> [Icw1_rms]
  Demux4/2 -> [Ibw1_rms]
  Demux4/1 -> [Iaw1_rms]
  Demux5/1 -> [Va_rms]
  Demux5/2 -> [Vb_rms]
  Demux5/3 -> [Vc_rms]
  Demux2/1 -> Fcn/1
  Fcn/1 -> 50/51 Relays 06122015/2
  [Iabc_w1] -> 50/51 Relays 06122015/1
  50/51 Relays 06122015/1 -> Logical Operator/1
  [Ibw1_mag] -> Bus Creator1/3
  [Icw1_mag] -> Bus Creator1/5
  [Va_mag] -> Bus Creator1/7
  [Vb_mag] -> Bus Creator1/9
  [Vc_mag] -> Bus Creator1/11
  Gain10/1 -> Bus Creator1/13
  Gain6/1 -> Bus Creator1/14
  Gain7/1 -> Bus Creator1/15
  [Iaw1_rms] -> Bus Creator1/18
  [Icw1_rms] -> Bus Creator1/20
  [Ibw1_rms] -> Bus Creator1/19
  [Va_rms] -> Bus Creator1/21
  [Vb_rms] -> Bus Creator1/22
  [Vc_rms] -> Bus Creator1/23
  Logical Operator/1 -> Logic_trip/1
  Demux2/2 -> op_mode/1
  [Iaw1_phase] -> Bus Creator1/2
  [Ibw1_phase] -> Bus Creator1/4
  [Icw1_phase] -> Bus Creator1/6
  [Va_phase] -> Bus Creator1/8
  [Vb_phase] -> Bus Creator1/10
  [Vb_phase] -> Bus Creator1/12
  Constant/1 -> Bus Creator1/24
  Constant1/1 -> Bus Creator1/25
  [Vabc] -> Gain2/1
  Gain2/1 -> Demux/1
  [Iabc_w1] -> Gain3/1
  Gain3/1 -> ?
  Demux10/1 -> [Va_mag]
  Demux10/2 -> [Vb_mag]
  Demux10/3 -> [Vc_mag]
  Complex to Magnitude-Angle/1 -> Demux10/1
  [Vabc] -> Complex to Magnitude-Angle/1
  Complex to Magnitude-Angle1/1 -> Demux11/1
  [Iabc_w1] -> Complex to Magnitude-Angle1/1
  Demux11/1 -> [Iaw1_mag]
  Demux11/2 -> [Ibw1_mag]
  Demux11/3 -> [Icw1_mag]

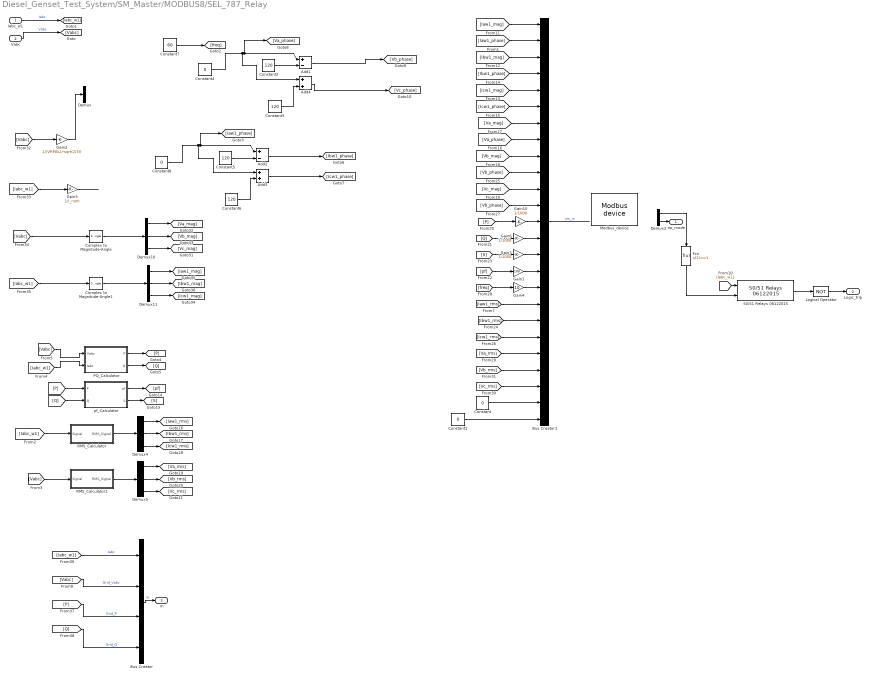
== system Diesel_Genset_Test_System/SM_Master/MODBUS8/SEL_787_Relay ==
  Iabc_w1 : Inport
  Vabc : Inport  Port=2
  50/51 Relays 06122015 : breakers_1ph_3ph/50//51 Relays 06122015  TOC=TOC  IOC=IOC  Ts=Ts
  Add1 : Sum  Inputs=+-
  Add2 : Sum  Inputs=+-
  Add3 : Sum
  Add4 : Sum
  Bus Creator : BusCreator
  Bus Creator1 : BusCreator  Inputs=25
  Complex to Magnitude-Angle : ComplexToMagnitudeAngle  Output=Magnitude
  Complex to Magnitude-Angle1 : ComplexToMagnitudeAngle  Output=Magnitude
  Constant{,1,4,8} (4 alike) : Constant  Value=0
  Constant{2..3,5..6} (4 alike) : Constant  Value=120
  Constant7 : Constant  Value=60
  Demux{,4..5,10..11} (5 alike) : Demux  Outputs=3
  Demux2 : Demux  Outputs=2
  Fcn : Fcn  Expr=u(1)==1
  Gain1 : Gain  Gain=100
  Gain10 : Gain  Gain=1/1000
  Gain2 : Gain  Gain=1/(VRMSLL*sqrt(2/3))
  Gain3 : Gain  Gain=1/I_nom
  Gain4 : Gain  Gain=10
  Gain6 : Gain  Gain=1/1000
  Gain7 : Gain  Gain=1/1000
  Logical Operator : Logic  Operator=NOT  AllPortsSameDT=off  OutDataTypeStr=boolean
  Modbus_device : rtio_generic_modbus/Modbus device  conf_name=none  conf_name_mask=relay_slave_cfg8.xls  sample_time=Ts
  PQ_Calculator : Subsystem
  RMS_Calculator : Subsystem
  RMS_Calculator1 : Subsystem
  pf_Calculator : Subsystem
  op_mode : Outport
  Logic_trip : Outport  Port=2
  m : Outport  Port=3
  wires:
  Gain4/1 -> Bus Creator1/17
  Gain1/1 -> Bus Creator1/16
  [pf] -> Gain1/1
  [freq] -> Gain4/1
  Constant4/1 -> Add4/1, [Va_phase], Add1/1
  Add4/1 -> [Vc_phase]
  Add1/1 -> [Vb_phase]
  Constant3/1 -> Add4/2
  Constant2/1 -> Add1/2
  Constant8/1 -> Add3/1, [Iaw1_phase], Add2/1
  Add3/1 -> [Icw1_phase]
  Add2/1 -> [Ibw1_phase]
  Constant6/1 -> Add3/2
  Constant5/1 -> Add2/2
  Constant7/1 -> [freq]
  pf_Calculator/2(S) -> [S]
  Bus Creator1/1 -> ?  "sm_in"
  ? -> Demux2/1
  [Q] -> Bus Creator/4  "Grid_Q"
  [P] -> Bus Creator/3  "Grid_P"
  [Vabc] -> Bus Creator/2  "Grid_Vabc"
  [Iabc_w1] -> Bus Creator/1  "Iabc"
  Bus Creator/1 -> m/1  "m"
  Iabc_w1/1 -> [Iabc_w1]  "Iabc"
  Vabc/1 -> [Vabc]  "Vabc"
  [Vabc] -> PQ_Calculator/1(Vabc)
  [Iabc_w1] -> PQ_Calculator/2(Iabc)
  [Iaw1_mag] -> Bus Creator1/1
  [P] -> Gain10/1
  [Q] -> Gain6/1
  [S] -> Gain7/1
  pf_Calculator/1(pf) -> [pf]
  [P] -> pf_Calculator/1(P)
  [Q] -> pf_Calculator/2(Q)
  PQ_Calculator/1(P) -> [P]
  PQ_Calculator/2(Q) -> [Q]
  [Iabc_w1] -> RMS_Calculator/1(Signal)
  [Vabc] -> RMS_Calculator1/1(Signal)
  RMS_Calculator/1(RMS_Signal) -> Demux4/1
  RMS_Calculator1/1(RMS_Signal) -> Demux5/1
  Demux4/3 -> [Icw1_rms]
  Demux4/2 -> [Ibw1_rms]
  Demux4/1 -> [Iaw1_rms]
  Demux5/1 -> [Va_rms]
  Demux5/2 -> [Vb_rms]
  Demux5/3 -> [Vc_rms]
  Demux2/1 -> Fcn/1
  Fcn/1 -> 50/51 Relays 06122015/2
  [Iabc_w1] -> 50/51 Relays 06122015/1
  50/51 Relays 06122015/1 -> Logical Operator/1
  [Ibw1_mag] -> Bus Creator1/3
  [Icw1_mag] -> Bus Creator1/5
  [Va_mag] -> Bus Creator1/7
  [Vb_mag] -> Bus Creator1/9
  [Vc_mag] -> Bus Creator1/11
  Gain10/1 -> Bus Creator1/13
  Gain6/1 -> Bus Creator1/14
  Gain7/1 -> Bus Creator1/15
  [Iaw1_rms] -> Bus Creator1/18
  [Icw1_rms] -> Bus Creator1/20
  [Ibw1_rms] -> Bus Creator1/19
  [Va_rms] -> Bus Creator1/21
  [Vb_rms] -> Bus Creator1/22
  [Vc_rms] -> Bus Creator1/23
  Logical Operator/1 -> Logic_trip/1
  Demux2/2 -> op_mode/1
  [Iaw1_phase] -> Bus Creator1/2
  [Ibw1_phase] -> Bus Creator1/4
  [Icw1_phase] -> Bus Creator1/6
  [Va_phase] -> Bus Creator1/8
  [Vb_phase] -> Bus Creator1/10
  [Vb_phase] -> Bus Creator1/12
  Constant/1 -> Bus Creator1/24
  Constant1/1 -> Bus Creator1/25
  [Vabc] -> Gain2/1
  Gain2/1 -> Demux/1
  [Iabc_w1] -> Gain3/1
  Gain3/1 -> ?
  Demux10/1 -> [Va_mag]
  Demux10/2 -> [Vb_mag]
  Demux10/3 -> [Vc_mag]
  Complex to Magnitude-Angle/1 -> Demux10/1
  [Vabc] -> Complex to Magnitude-Angle/1
  Complex to Magnitude-Angle1/1 -> Demux11/1
  [Iabc_w1] -> Complex to Magnitude-Angle1/1
  Demux11/1 -> [Iaw1_mag]
  Demux11/2 -> [Ibw1_mag]
  Demux11/3 -> [Icw1_mag]

== system Diesel_Genset_Test_System/SC_Console/Woodward/16TSDIn/16 TSDOut GR3/Din/Dout ch16-23 ==
  Bus Creator3 : BusCreator  Inputs=8
  times17 : Constant  Value=[0.05 0.15 0.25 0.35]
  times18 : Constant  Value=[0.1 0.2 0.3 0.4]
  times19 : Constant  Value=[0.15 0.25 0.35 0.45]
  times20 : Constant  Value=[0.2 0.3 0.4 0.5]
  times21 : Constant  Value=[0.25 0.35 0.45 0.55]
  times22 : Constant  Value=[0.3 0.4 0.5 0.6]
  times23 : Constant  Value=[0.3 0.4 0.5 0.6]
  times24 : Constant  Value=[0 0.1 0.2 0.3]
  Out1 : Outport
  wires:
  Bus Creator3/1 -> Out1/1
  times23/1 -> Bus Creator3/8  "times24"
  times22/1 -> Bus Creator3/7  "times23"
  times21/1 -> Bus Creator3/6  "times22"
  times20/1 -> Bus Creator3/5  "times21"
  times19/1 -> Bus Creator3/4  "times20"
  times18/1 -> Bus Creator3/3  "times19"
  times17/1 -> Bus Creator3/2  "times18"
  times24/1 -> Bus Creator3/1  "times17"

== system Diesel_Genset_Test_System/SC_Console/Woodward/16TSDIn/16 TSDOut GR3/Din/Dout ch24-31 ==
  Bus Creator4 : BusCreator  Inputs=8
  times25 : Constant  Value=[0.05 0.15 0.25 0.35]
  times26 : Constant  Value=[0.1 0.2 0.3 0.4]
  times27 : Constant  Value=[0.15 0.25 0.35 0.45]
  times28 : Constant  Value=[0.2 0.3 0.4 0.5]
  times29 : Constant  Value=[0.25 0.35 0.45 0.55]
  times30 : Constant  Value=[0.3 0.4 0.5 0.6]
  times31 : Constant  Value=[0.3 0.4 0.5 0.6]
  times32 : Constant  Value=[0 0.1 0.2 0.3]
  Out1 : Outport
  wires:
  Bus Creator4/1 -> Out1/1
  times31/1 -> Bus Creator4/8  "times32"
  times30/1 -> Bus Creator4/7  "times31"
  times29/1 -> Bus Creator4/6  "times30"
  times28/1 -> Bus Creator4/5  "times29"
  times27/1 -> Bus Creator4/4  "times28"
  times26/1 -> Bus Creator4/3  "times27"
  times25/1 -> Bus Creator4/2  "times26"
  times32/1 -> Bus Creator4/1  "times25"

== system Diesel_Genset_Test_System/SC_Console/Woodward/16TSDIn/16 TSDOut GR3/Dout state ctrl ==
  Bus Creator : BusCreator  Inputs=2
  Dout_CH16_CH23 : Subsystem
  Dout_CH24_CH31 : Subsystem
  Event State OUT : Outport
  wires:
  Dout_CH24_CH31/1(Dout_CH8_CH15) -> Bus Creator/2  "CH24-31"
  Dout_CH16_CH23/1(Dout_CH8_CH15) -> Bus Creator/1  "CH16-23"
  Bus Creator/1 -> Event State OUT/1

== system Diesel_Genset_Test_System/SM_Master/MODBUS1/SEL_787_Relay/PQ_Calculator ==
  Vabc : Inport
  Iabc : Inport  Port=2
  3-phase  Instantaneous  Active & Reactive Power : powerlib_extras/Measurements/3-phase  Instantaneous  Active & Reactive Power
  Demux : Demux  Outputs=2
  Discrete  Mean value2 : powerlib_extras/Discrete Measurements/Discrete  Mean value  Freq=60  Vinit=0  Ts=Ts
  P : Outport
  Q : Outport  Port=2
  wires:
  3-phase  Instantaneous  Active & Reactive Power/1 -> Discrete  Mean value2/1
  Discrete  Mean value2/1 -> Demux/1
  Vabc/1 -> 3-phase  Instantaneous  Active & Reactive Power/1
  Iabc/1 -> 3-phase  Instantaneous  Active & Reactive Power/2
  Demux/1 -> P/1  "P"
  Demux/2 -> Q/1  "Q"

== system Diesel_Genset_Test_System/SM_Master/MODBUS1/SEL_787_Relay/RMS_Calculator ==
  Signal : Inport
  Discrete  Mean value6 : powerlib_extras/Discrete Measurements/Discrete  Mean value  Freq=60  Vinit=0  Ts=Ts
  Product3 : Product  RndMeth=Zero
  Signed Sqrt : Sqrt  SaturateOnIntegerOverflow=on
  RMS_Signal : Outport
  wires:
  Signal/1 -> Product3/1, Product3/2
  Product3/1 -> Discrete  Mean value6/1
  Discrete  Mean value6/1 -> Signed Sqrt/1
  Signed Sqrt/1 -> RMS_Signal/1

== system Diesel_Genset_Test_System/SM_Master/MODBUS1/SEL_787_Relay/RMS_Calculator1 ==
  Signal : Inport
  Discrete  Mean value6 : powerlib_extras/Discrete Measurements/Discrete  Mean value  Freq=60  Vinit=0  Ts=Ts
  Product3 : Product  RndMeth=Zero
  Signed Sqrt : Sqrt  SaturateOnIntegerOverflow=on
  RMS_Signal : Outport
  wires:
  Signal/1 -> Product3/1, Product3/2
  Product3/1 -> Discrete  Mean value6/1
  Discrete  Mean value6/1 -> Signed Sqrt/1
  Signed Sqrt/1 -> RMS_Signal/1

== system Diesel_Genset_Test_System/SM_Master/MODBUS1/SEL_787_Relay/pf_Calculator ==
  P : Inport
  Q : Inport  Port=2
  Fcn : Fcn  Expr=u(1) / sqrt(u(1)^2 + u(2)^2)
  Fcn1 : Fcn  Expr=sqrt(u(1)^2 + u(2)^2)
  Mux : Mux  Inputs=2
  Mux1 : Mux  Inputs=2
  Scope : Scope
      settings: YMin=0.8475  YMax=0.875  SaveName=ScopeData2
  pf : Outport
  S : Outport  Port=2
  wires:
  Fcn1/1 -> S/1
  Mux1/1 -> Fcn1/1
  Fcn/1 -> Scope/1, pf/1
  Mux/1 -> Fcn/1
  P/1 -> Mux1/1, Mux/1
  Q/1 -> Mux1/2, Mux/2

== system Diesel_Genset_Test_System/SM_Master/MODBUS2/SEL_787_Relay/PQ_Calculator ==
  Vabc : Inport
  Iabc : Inport  Port=2
  3-phase  Instantaneous  Active & Reactive Power : powerlib_extras/Measurements/3-phase  Instantaneous  Active & Reactive Power
  Demux : Demux  Outputs=2
  Discrete  Mean value2 : powerlib_extras/Discrete Measurements/Discrete  Mean value  Freq=60  Vinit=0  Ts=Ts
  P : Outport
  Q : Outport  Port=2
  wires:
  3-phase  Instantaneous  Active & Reactive Power/1 -> Discrete  Mean value2/1
  Discrete  Mean value2/1 -> Demux/1
  Vabc/1 -> 3-phase  Instantaneous  Active & Reactive Power/1
  Iabc/1 -> 3-phase  Instantaneous  Active & Reactive Power/2
  Demux/1 -> P/1  "P"
  Demux/2 -> Q/1  "Q"

== system Diesel_Genset_Test_System/SM_Master/MODBUS2/SEL_787_Relay/RMS_Calculator ==
  Signal : Inport
  Discrete  Mean value6 : powerlib_extras/Discrete Measurements/Discrete  Mean value  Freq=60  Vinit=0  Ts=Ts
  Product3 : Product  RndMeth=Zero
  Signed Sqrt : Sqrt  SaturateOnIntegerOverflow=on
  RMS_Signal : Outport
  wires:
  Signal/1 -> Product3/1, Product3/2
  Product3/1 -> Discrete  Mean value6/1
  Discrete  Mean value6/1 -> Signed Sqrt/1
  Signed Sqrt/1 -> RMS_Signal/1

== system Diesel_Genset_Test_System/SM_Master/MODBUS2/SEL_787_Relay/RMS_Calculator1 ==
  Signal : Inport
  Discrete  Mean value6 : powerlib_extras/Discrete Measurements/Discrete  Mean value  Freq=60  Vinit=0  Ts=Ts
  Product3 : Product  RndMeth=Zero
  Signed Sqrt : Sqrt  SaturateOnIntegerOverflow=on
  RMS_Signal : Outport
  wires:
  Signal/1 -> Product3/1, Product3/2
  Product3/1 -> Discrete  Mean value6/1
  Discrete  Mean value6/1 -> Signed Sqrt/1
  Signed Sqrt/1 -> RMS_Signal/1

== system Diesel_Genset_Test_System/SM_Master/MODBUS2/SEL_787_Relay/pf_Calculator ==
  P : Inport
  Q : Inport  Port=2
  Fcn : Fcn  Expr=u(1) / sqrt(u(1)^2 + u(2)^2)
  Fcn1 : Fcn  Expr=sqrt(u(1)^2 + u(2)^2)
  Mux : Mux  Inputs=2
  Mux1 : Mux  Inputs=2
  Scope : Scope
      settings: YMin=0.8475  YMax=0.875  SaveName=ScopeData2
  pf : Outport
  S : Outport  Port=2
  wires:
  Fcn1/1 -> S/1
  Mux1/1 -> Fcn1/1
  Fcn/1 -> Scope/1, pf/1
  Mux/1 -> Fcn/1
  P/1 -> Mux1/1, Mux/1
  Q/1 -> Mux1/2, Mux/2

== system Diesel_Genset_Test_System/SM_Master/MODBUS4/SEL_787_Relay/PQ_Calculator ==
  Vabc : Inport
  Iabc : Inport  Port=2
  3-phase  Instantaneous  Active & Reactive Power : powerlib_extras/Measurements/3-phase  Instantaneous  Active & Reactive Power
  Demux : Demux  Outputs=2
  Discrete  Mean value2 : powerlib_extras/Discrete Measurements/Discrete  Mean value  Freq=60  Vinit=0  Ts=Ts
  P : Outport
  Q : Outport  Port=2
  wires:
  3-phase  Instantaneous  Active & Reactive Power/1 -> Discrete  Mean value2/1
  Discrete  Mean value2/1 -> Demux/1
  Vabc/1 -> 3-phase  Instantaneous  Active & Reactive Power/1
  Iabc/1 -> 3-phase  Instantaneous  Active & Reactive Power/2
  Demux/1 -> P/1  "P"
  Demux/2 -> Q/1  "Q"

== system Diesel_Genset_Test_System/SM_Master/MODBUS4/SEL_787_Relay/RMS_Calculator ==
  Signal : Inport
  Discrete  Mean value6 : powerlib_extras/Discrete Measurements/Discrete  Mean value  Freq=60  Vinit=0  Ts=Ts
  Product3 : Product  RndMeth=Zero
  Signed Sqrt : Sqrt  SaturateOnIntegerOverflow=on
  RMS_Signal : Outport
  wires:
  Signal/1 -> Product3/1, Product3/2
  Product3/1 -> Discrete  Mean value6/1
  Discrete  Mean value6/1 -> Signed Sqrt/1
  Signed Sqrt/1 -> RMS_Signal/1

== system Diesel_Genset_Test_System/SM_Master/MODBUS4/SEL_787_Relay/RMS_Calculator1 ==
  Signal : Inport
  Discrete  Mean value6 : powerlib_extras/Discrete Measurements/Discrete  Mean value  Freq=60  Vinit=0  Ts=Ts
  Product3 : Product  RndMeth=Zero
  Signed Sqrt : Sqrt  SaturateOnIntegerOverflow=on
  RMS_Signal : Outport
  wires:
  Signal/1 -> Product3/1, Product3/2
  Product3/1 -> Discrete  Mean value6/1
  Discrete  Mean value6/1 -> Signed Sqrt/1
  Signed Sqrt/1 -> RMS_Signal/1

== system Diesel_Genset_Test_System/SM_Master/MODBUS4/SEL_787_Relay/pf_Calculator ==
  P : Inport
  Q : Inport  Port=2
  Fcn : Fcn  Expr=u(1) / sqrt(u(1)^2 + u(2)^2)
  Fcn1 : Fcn  Expr=sqrt(u(1)^2 + u(2)^2)
  Mux : Mux  Inputs=2
  Mux1 : Mux  Inputs=2
  Scope : Scope
      settings: YMin=0.8475  YMax=0.875  SaveName=ScopeData2
  pf : Outport
  S : Outport  Port=2
  wires:
  Fcn1/1 -> S/1
  Mux1/1 -> Fcn1/1
  Fcn/1 -> Scope/1, pf/1
  Mux/1 -> Fcn/1
  P/1 -> Mux1/1, Mux/1
  Q/1 -> Mux1/2, Mux/2

== system Diesel_Genset_Test_System/SM_Master/MODBUS5/SEL_787_Relay/PQ_Calculator ==
  Vabc : Inport
  Iabc : Inport  Port=2
  3-phase  Instantaneous  Active & Reactive Power : powerlib_extras/Measurements/3-phase  Instantaneous  Active & Reactive Power
  Demux : Demux  Outputs=2
  Discrete  Mean value2 : powerlib_extras/Discrete Measurements/Discrete  Mean value  Freq=60  Vinit=0  Ts=Ts
  P : Outport
  Q : Outport  Port=2
  wires:
  3-phase  Instantaneous  Active & Reactive Power/1 -> Discrete  Mean value2/1
  Discrete  Mean value2/1 -> Demux/1
  Vabc/1 -> 3-phase  Instantaneous  Active & Reactive Power/1
  Iabc/1 -> 3-phase  Instantaneous  Active & Reactive Power/2
  Demux/1 -> P/1  "P"
  Demux/2 -> Q/1  "Q"

== system Diesel_Genset_Test_System/SM_Master/MODBUS5/SEL_787_Relay/RMS_Calculator ==
  Signal : Inport
  Discrete  Mean value6 : powerlib_extras/Discrete Measurements/Discrete  Mean value  Freq=60  Vinit=0  Ts=Ts
  Product3 : Product  RndMeth=Zero
  Signed Sqrt : Sqrt  SaturateOnIntegerOverflow=on
  RMS_Signal : Outport
  wires:
  Signal/1 -> Product3/1, Product3/2
  Product3/1 -> Discrete  Mean value6/1
  Discrete  Mean value6/1 -> Signed Sqrt/1
  Signed Sqrt/1 -> RMS_Signal/1

== system Diesel_Genset_Test_System/SM_Master/MODBUS5/SEL_787_Relay/RMS_Calculator1 ==
  Signal : Inport
  Discrete  Mean value6 : powerlib_extras/Discrete Measurements/Discrete  Mean value  Freq=60  Vinit=0  Ts=Ts
  Product3 : Product  RndMeth=Zero
  Signed Sqrt : Sqrt  SaturateOnIntegerOverflow=on
  RMS_Signal : Outport
  wires:
  Signal/1 -> Product3/1, Product3/2
  Product3/1 -> Discrete  Mean value6/1
  Discrete  Mean value6/1 -> Signed Sqrt/1
  Signed Sqrt/1 -> RMS_Signal/1

== system Diesel_Genset_Test_System/SM_Master/MODBUS5/SEL_787_Relay/pf_Calculator ==
  P : Inport
  Q : Inport  Port=2
  Fcn : Fcn  Expr=u(1) / sqrt(u(1)^2 + u(2)^2)
  Fcn1 : Fcn  Expr=sqrt(u(1)^2 + u(2)^2)
  Mux : Mux  Inputs=2
  Mux1 : Mux  Inputs=2
  Scope : Scope
      settings: YMin=0.8475  YMax=0.875  SaveName=ScopeData2
  pf : Outport
  S : Outport  Port=2
  wires:
  Fcn1/1 -> S/1
  Mux1/1 -> Fcn1/1
  Fcn/1 -> Scope/1, pf/1
  Mux/1 -> Fcn/1
  P/1 -> Mux1/1, Mux/1
  Q/1 -> Mux1/2, Mux/2

== system Diesel_Genset_Test_System/SM_Master/MODBUS6/SEL_787_Relay/PQ_Calculator ==
  Vabc : Inport
  Iabc : Inport  Port=2
  3-phase  Instantaneous  Active & Reactive Power : powerlib_extras/Measurements/3-phase  Instantaneous  Active & Reactive Power
  Demux : Demux  Outputs=2
  Discrete  Mean value2 : powerlib_extras/Discrete Measurements/Discrete  Mean value  Freq=60  Vinit=0  Ts=Ts
  P : Outport
  Q : Outport  Port=2
  wires:
  3-phase  Instantaneous  Active & Reactive Power/1 -> Discrete  Mean value2/1
  Discrete  Mean value2/1 -> Demux/1
  Vabc/1 -> 3-phase  Instantaneous  Active & Reactive Power/1
  Iabc/1 -> 3-phase  Instantaneous  Active & Reactive Power/2
  Demux/1 -> P/1  "P"
  Demux/2 -> Q/1  "Q"

== system Diesel_Genset_Test_System/SM_Master/MODBUS6/SEL_787_Relay/RMS_Calculator ==
  Signal : Inport
  Discrete  Mean value6 : powerlib_extras/Discrete Measurements/Discrete  Mean value  Freq=60  Vinit=0  Ts=Ts
  Product3 : Product  RndMeth=Zero
  Signed Sqrt : Sqrt  SaturateOnIntegerOverflow=on
  RMS_Signal : Outport
  wires:
  Signal/1 -> Product3/1, Product3/2
  Product3/1 -> Discrete  Mean value6/1
  Discrete  Mean value6/1 -> Signed Sqrt/1
  Signed Sqrt/1 -> RMS_Signal/1

== system Diesel_Genset_Test_System/SM_Master/MODBUS6/SEL_787_Relay/RMS_Calculator1 ==
  Signal : Inport
  Discrete  Mean value6 : powerlib_extras/Discrete Measurements/Discrete  Mean value  Freq=60  Vinit=0  Ts=Ts
  Product3 : Product  RndMeth=Zero
  Signed Sqrt : Sqrt  SaturateOnIntegerOverflow=on
  RMS_Signal : Outport
  wires:
  Signal/1 -> Product3/1, Product3/2
  Product3/1 -> Discrete  Mean value6/1
  Discrete  Mean value6/1 -> Signed Sqrt/1
  Signed Sqrt/1 -> RMS_Signal/1

== system Diesel_Genset_Test_System/SM_Master/MODBUS6/SEL_787_Relay/pf_Calculator ==
  P : Inport
  Q : Inport  Port=2
  Fcn : Fcn  Expr=u(1) / sqrt(u(1)^2 + u(2)^2)
  Fcn1 : Fcn  Expr=sqrt(u(1)^2 + u(2)^2)
  Mux : Mux  Inputs=2
  Mux1 : Mux  Inputs=2
  Scope : Scope
      settings: YMin=0.8475  YMax=0.875  SaveName=ScopeData2
  pf : Outport
  S : Outport  Port=2
  wires:
  Fcn1/1 -> S/1
  Mux1/1 -> Fcn1/1
  Fcn/1 -> Scope/1, pf/1
  Mux/1 -> Fcn/1
  P/1 -> Mux1/1, Mux/1
  Q/1 -> Mux1/2, Mux/2

== system Diesel_Genset_Test_System/SM_Master/MODBUS8/SEL_787_Relay/PQ_Calculator ==
  Vabc : Inport
  Iabc : Inport  Port=2
  3-phase  Instantaneous  Active & Reactive Power : powerlib_extras/Measurements/3-phase  Instantaneous  Active & Reactive Power
  Demux : Demux  Outputs=2
  Discrete  Mean value2 : powerlib_extras/Discrete Measurements/Discrete  Mean value  Freq=60  Vinit=0  Ts=Ts
  P : Outport
  Q : Outport  Port=2
  wires:
  3-phase  Instantaneous  Active & Reactive Power/1 -> Discrete  Mean value2/1
  Discrete  Mean value2/1 -> Demux/1
  Vabc/1 -> 3-phase  Instantaneous  Active & Reactive Power/1
  Iabc/1 -> 3-phase  Instantaneous  Active & Reactive Power/2
  Demux/1 -> P/1  "P"
  Demux/2 -> Q/1  "Q"

== system Diesel_Genset_Test_System/SM_Master/MODBUS8/SEL_787_Relay/RMS_Calculator ==
  Signal : Inport
  Discrete  Mean value6 : powerlib_extras/Discrete Measurements/Discrete  Mean value  Freq=60  Vinit=0  Ts=Ts
  Product3 : Product  RndMeth=Zero
  Signed Sqrt : Sqrt  SaturateOnIntegerOverflow=on
  RMS_Signal : Outport
  wires:
  Signal/1 -> Product3/1, Product3/2
  Product3/1 -> Discrete  Mean value6/1
  Discrete  Mean value6/1 -> Signed Sqrt/1
  Signed Sqrt/1 -> RMS_Signal/1

== system Diesel_Genset_Test_System/SM_Master/MODBUS8/SEL_787_Relay/RMS_Calculator1 ==
  Signal : Inport
  Discrete  Mean value6 : powerlib_extras/Discrete Measurements/Discrete  Mean value  Freq=60  Vinit=0  Ts=Ts
  Product3 : Product  RndMeth=Zero
  Signed Sqrt : Sqrt  SaturateOnIntegerOverflow=on
  RMS_Signal : Outport
  wires:
  Signal/1 -> Product3/1, Product3/2
  Product3/1 -> Discrete  Mean value6/1
  Discrete  Mean value6/1 -> Signed Sqrt/1
  Signed Sqrt/1 -> RMS_Signal/1

== system Diesel_Genset_Test_System/SM_Master/MODBUS8/SEL_787_Relay/pf_Calculator ==
  P : Inport
  Q : Inport  Port=2
  Fcn : Fcn  Expr=u(1) / sqrt(u(1)^2 + u(2)^2)
  Fcn1 : Fcn  Expr=sqrt(u(1)^2 + u(2)^2)
  Mux : Mux  Inputs=2
  Mux1 : Mux  Inputs=2
  Scope : Scope
      settings: YMin=0.8475  YMax=0.875  SaveName=ScopeData2
  pf : Outport
  S : Outport  Port=2
  wires:
  Fcn1/1 -> S/1
  Mux1/1 -> Fcn1/1
  Fcn/1 -> Scope/1, pf/1
  Mux/1 -> Fcn/1
  P/1 -> Mux1/1, Mux/1
  Q/1 -> Mux1/2, Mux/2
